simulink model "PIDRegler"  (R2023a)
settings: Solver=VariableStepAuto  StartTime=0.0  StopTime=inf  FixedStep=1/30  RelTol=1e-3
undefined symbols (not defined in the file or in its folder): DiscIntNeverNeededParam, gray, LF, none, videoinput
libraries: instrumentseriallib x3, visiontextngfix x1, svdutilitieslib x1, imaqlib x1, simulink_extras x1, simulink x1
settings Model: Creator=Legenden-PC  LastModifiedBy=Legenden-PC
settings OptimizationCC: ReuseModelBlockBuffer=off

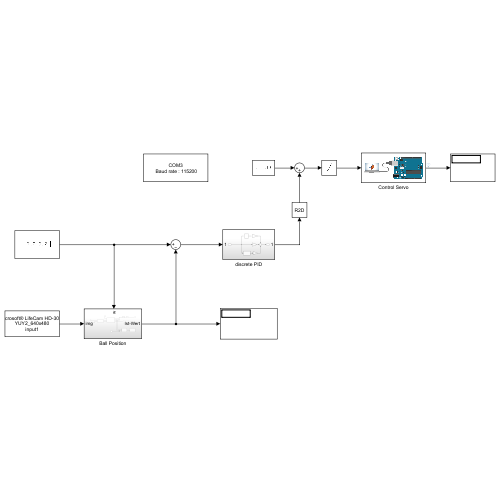
[thumbnail: Simulink's stored preview of the top-level diagram]
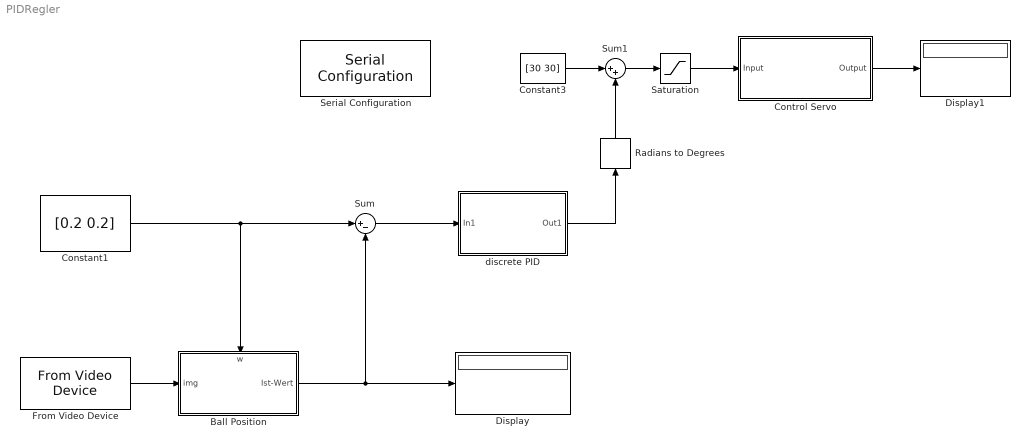
== system PIDRegler ==
  Ball Position : Subsystem
      settings: PortSchema="{\"entries\":[{\"content\":{\"sides\":[{\"content\":{\"connectorIds\":[\"In1\"]},\"type\":\"ConnectorPlacement.EquallySpacedRectSide\",\"uuid\":\"ceb15f42-21bb-4f4e-b2bb-f76c0e940da7\"},{\"content\":{\"connectorIds\":[\"Out1\"],\"side\":\"RIGHT\"},\"type\":\"ConnectorPlacement.EquallySpacedRectSide\",\"uuid\":\"4847c9c9-69f0-4792-8281-833646641724\"},{\"content\":{\"connectorIds\":[\"In2\"],\"side\":\"TOP\"},\"type\":\"ConnectorPlacement.EquallySpacedRectSide\",\"uuid\":\"e3feb0c1-2393-47b7-9586-54aa1cda8109\"}]},\"type\":\"ConnectorPlacement.EquallySpacedConnector\",\"uuid\":\"4d95092f-21d8-4983-983f-3a93ab7da789\"}],\"packageUris\":[\"http://schema.mathworks.com/mf0/Connector/R2020b\"],\"version\":\"1.0\"}"
  Constant1 : Constant  Value=[0.2 0.2]  VectorParams1D=off  SampleTime=1/30
  Constant3 : Constant  Value=[30 30]
  Control Servo : Subsystem
      mask Display: image('C:\Users\Legenden-PC\Desktop\arduino_usb.png'); % Use "Edit Image" on toolstrip to change.
  Display : Display
  Display1 : Display
  From Video Device : imaqlib/From Video Device  DeviceMenu=winvideo 1 (Iriun Webcam)  Device=winvideo 1 (Microsoft® LifeCam HD-3000)  ObjConstructor=videoinput('winvideo', 1)  VideoFormatMenu=YUY2_640x480  VideoFormat=YUY2_640x480  VideoSource=input1  ROIPosition=[0 0 480 640]  EnableHWTrigger=off  TriggerConfiguration=none/none  SampleTime=1/30  OutputPortsMode=One multidimensional signal  DataType=single  CanDoHWTrigger=no  ReturnedColorSpace=rgb  BlockHandle=140.0005  ROIWidth=640  ROIHeight=480  ROIColumn=0  ROIRow=0  EngXMLPath=C:\Program Files\MATLAB\R2023a\toolbox\imaq\imaq\private  DevXMLPath=C:\ProgramData\MATLAB\SupportPackages\R2023a\toolbox\imaq\supportpackages\genericvideo\adaptor\win64  EngLibPath=C:\Program Files\MATLAB\R2023a\toolbox\imaq\imaqblks\imaqmex\win64  ColorSpace=rgb  BayerSensorAlignment=grbg  ImaqMode=off
  Radians to Degrees : simulink_extras/Transformations/Radians to Degrees
  Saturation : Saturate  UpperLimit=50  LowerLimit=10
  Serial Configuration : instrumentseriallib/Serial Configuration  Priority=-200000  PortSel=COM3  Port=COM3  ComPort=COM3  BaudRate=115200  DataBits=8  Parity=none  StopBits=1  ByteOrder=little-endian  FlowControl=none  Timeout=10  SimulateUsing=Interpreted execution  BlockInModel=on  aMode=1
  Sum : Sum  Inputs=|+-
  Sum1 : Sum  Inputs=|++
  discrete PID : Subsystem
  wires:
  Saturation/1 -> Control Servo/1(Input)
  Sum1/1 -> Saturation/1
  Control Servo/1(Output) -> Display1/1
  Constant3/1 -> Sum1/1
  Radians to Degrees/1 -> Sum1/2
  Constant1/1 -> Ball Position/2(w), Sum/1
  Sum/1 -> discrete PID/1(In1)
  discrete PID/1(Out1) -> Radians to Degrees/1
  Ball Position/1(Ist-Wert) -> Sum/2, Display/1
  From Video Device/1 -> Ball Position/1("img ")

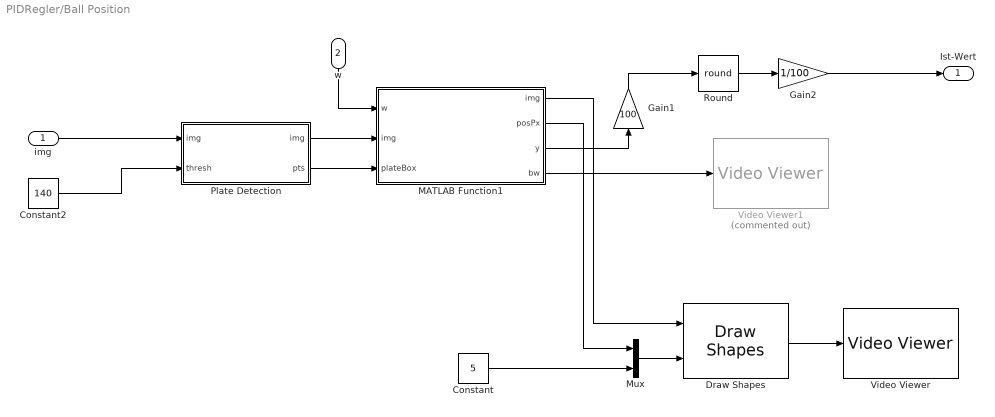
== system PIDRegler/Ball Position ==
  "img " : Inport
  w : Inport  Port=2
  Constant : Constant  Value=5  VectorParams1D=off
  Constant2 : Constant  Value=140
  Draw Shapes : visiontextngfix/Draw Shapes  shape=Circles  fill=off  lineWidth=3  fillClrSource=Specify via dialog  display=Black  intensity=200  color=[200 255 100]  opacity=0.6  viewport=Entire image  antialiasing=off  inType=Obsolete  imagePorts=One multidimensional signal  roundingMode=Floor  overflowMode=off  memoryMode=Specify word length  memoryWordLength=16  prodOutputMode=Binary point scaling  prodOutputWordLength=32  prodOutputFracLength=14  memoryFracLength=15
  Gain1 : Gain  Gain=100
  Gain2 : Gain  Gain=1/100
  MATLAB Function1 : MATLAB Function  TreatAsAtomicUnit=on
  Mux : Mux  Inputs=2
  Plate Detection : MATLAB Function  TreatAsAtomicUnit=on
  Round : Rounding  Operator=round
  Video Viewer : VideoViewer  colormapValue=gray(256)  FigPos=[1031 805 816 339]
  Video Viewer1 : VideoViewer  Commented=on  FigPos=[179 908 614 489]
  Ist-Wert : Outport
  wires:
  MATLAB Function1/4(bw) -> Video Viewer1/1
  Plate Detection/1(img) -> MATLAB Function1/2("img ")
  Round/1 -> Gain2/1
  Gain1/1 -> Round/1
  Constant/1 -> Mux/2
  Mux/1 -> Draw Shapes/2
  MATLAB Function1/2(posPx) -> Mux/1
  Plate Detection/2(pts) -> MATLAB Function1/3(plateBox)
  Constant2/1 -> Plate Detection/2(thresh)
  MATLAB Function1/3(y) -> Gain1/1
  Draw Shapes/1 -> Video Viewer/1
  MATLAB Function1/1(img) -> Draw Shapes/1
  Gain2/1 -> Ist-Wert/1
  "img "/1 -> Plate Detection/1("img ")
  w/1 -> MATLAB Function1/1(w)

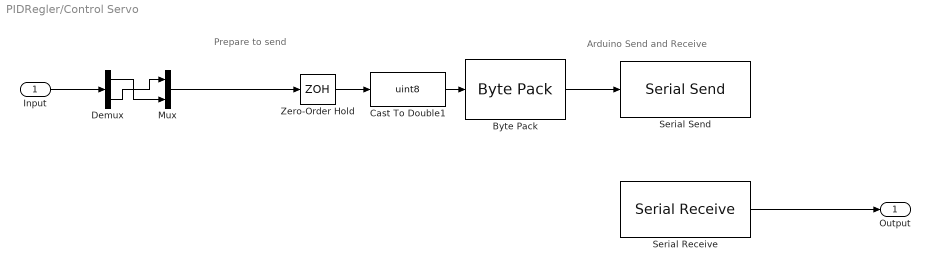
== system PIDRegler/Control Servo ==
  note: Prepare to send
  note: Arduino Send and Receive
  Input : Inport
  Byte Pack : svdutilitieslib/Byte Pack  maskPackedDataType=uint8  datatypes={'uint8'}  byteAlign=2  blockPlatform=arduinoert
  Cast To Double1 : DataTypeConversion  OutDataTypeStr=uint8  SaturateOnIntegerOverflow=off  RndMeth=Floor
  Demux : Demux  Outputs=2
  Mux : Mux  Inputs=2
  Serial Receive : instrumentseriallib/Serial Receive  PortSel=COM3  Port=COM3  ComPort=COM3  DataType=uint8  SaveDataType=uint8  ToggleHeader=on  Header=[ 65 ]  ToggleTerminator=on  Terminator=LF ('\n')  CustomTerminator=[]  InputFormat=Column major  ToggleDataSize=on  DataSize="[1  2]"  EnableBlockingMode=on  ActionDataUnavailable=Output last received value  ActionWhenDataUnavailable=Output last received value  CustomValue=0  SampleTime=0.01  SimulateUsing=Interpreted execution  BlockInModel=on  aMode=1
  Serial Send : instrumentseriallib/Serial Send  PortSel=COM3  Port=COM3  ComPort=COM3  Header=[]  Terminator=<none>  CustomTerminator=[]  EnableBlockingMode=on  SimulateUsing=Interpreted execution  BlockInModel=on  aMode=1
  Zero-Order Hold : ZeroOrderHold  SampleTime=0.01
  Output : Outport
  wires:
  Cast To Double1/1 -> Byte Pack/1
  Byte Pack/1 -> Serial Send/1
  Serial Receive/1 -> Output/1
  Zero-Order Hold/1 -> Cast To Double1/1
  Input/1 -> Demux/1
  Demux/1 -> Mux/2
  Demux/2 -> Mux/1
  Mux/1 -> Zero-Order Hold/1

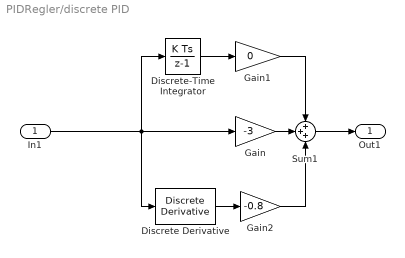
== system PIDRegler/discrete PID ==
  In1 : Inport
  Discrete Derivative : simulink/Discrete/Discrete Derivative  gainval=1.0  ICPrevScaledInput=0.0  OutMin=[]  OutMax=[]  OutDataType=fixdt(1, 16)  OutScaling=2^-10  DoSatur=off
  Discrete-Time Integrator : DiscreteIntegrator  SampleTime=1/30  ICPrevOutput=DiscIntNeverNeededParam  ICPrevScaledInput=DiscIntNeverNeededParam
  Gain : Gain  Gain=-3
  Gain1 : Gain  Gain=0
  Gain2 : Gain  Gain=-0.8
  Sum1 : Sum  Inputs=+++
  Out1 : Outport
  wires:
  Gain/1 -> Sum1/2
  Gain2/1 -> Sum1/3
  Discrete Derivative/1 -> Gain2/1
  Discrete-Time Integrator/1 -> Gain1/1
  Gain1/1 -> Sum1/1
  Sum1/1 -> Out1/1
  In1/1 -> Discrete Derivative/1, Discrete-Time Integrator/1, Gain/1

== matlab function PIDRegler/Ball Position/MATLAB Function1 ==
  data: w input; img input; img output size=480,640; plateBox input; posPx output; y output; bw output size=640,640
function [img, posPx, y, bw] = ballDetection(w,img, plateBox)

    persistent Hblob  prevPos
    
    
    plateBox = double(plateBox);

    if isempty(Hblob)
       Hblob = vision.BlobAnalysis('PerimeterOutputPort',1,'MinimumBlobArea',1500,'MaximumBlobArea',3300,'MaximumCount',10);
       prevPos =  zeros(1,2);
    end
    
    if ~isequal(plateBox,zeros(1,4))
        bw = rgb2gray(imcrop(img,plateBox))>150/255;                                %rgb2gray(imcrop(img,plateBox))>230;
        [area,ct,~,perimeter] = Hblob(bw);
        pos = ct(4*pi*double(area)./(perimeter.^2)>0.8,1:2);
        
        
        if isempty(pos)
            posPx = prevPos(1,1:2);
            y = w;
        else 
            prevPos = pos(1,1:2)+plateBox(1:2);
            posPx = prevPos(1,1:2);
            y = (posPx-plateBox(1:2)).*0.4./[plateBox(3) plateBox(4)];
        end
        
        
    else
        posPx = zeros(1,2,"double");
        y = w;
        bw = rgb2gray(img)>150/255;
    end
end

== matlab function PIDRegler/Ball Position/Plate Detection ==
  data: img output; img input; pts output; thresh input
function [img,pts] = getPlatePts(img,thresh)

persistent bbox

    

if isempty(bbox)
    hBlob = vision.BlobAnalysis('AreaOutputPort',1, ...
                                'BoundingBoxOutputPort',1, ...
                                'ExcludeBorderBlobs',0, ...
                                'MinimumBlobArea',450^2,...
                                'MaximumBlobArea',490^2);
    grayimg = im2gray(img);
    bw = grayimg < thresh/255;
    
    bw = imerode(bw,strel("square",8));
    
    [~,~,bbox ] = hBlob(bw);
end

if isempty(bbox)
    pts = zeros(1,4,"int32");
else
    pts = [bbox(1,1)+10 bbox(1,2) 480 480];
end
